simulink model "bai5"  (R2023a)
settings: Solver=VariableStepAuto  StartTime=0.0  StopTime=10.0  RelTol=1e-3
libraries: commdigbbndam3 x4, dspxfrm3 x3, eeGeneralControl x3, commchan3 x2, commsink2 x2, dspsigattribs x1, dspspect3 x1, commrflib2 x1, commrandsrc3 x1, dspstat3 x1
settings Model: Creator=USER  LastModifiedBy=Admin

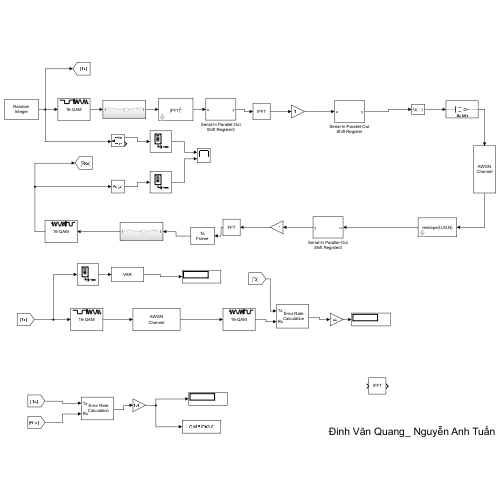
[thumbnail: Simulink's stored preview of the top-level diagram]
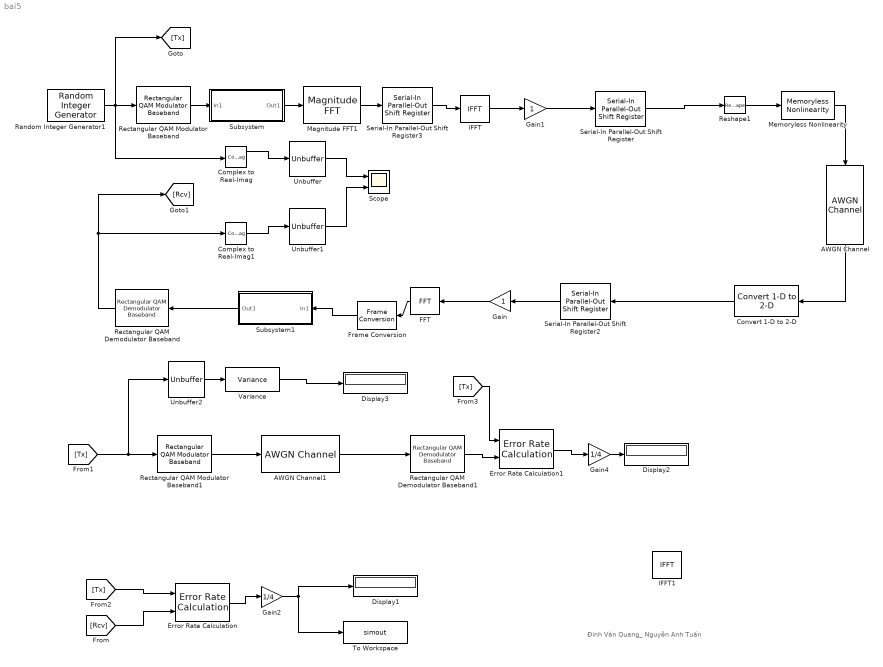
== system bai5 ==
  note: Đinh Văn Quang_ Nguyễn Anh Tuấn
  AWGN Channel : commchan3/AWGN Channel  LegacyMode=off  NoiseMethod="Signal to noise ratio  (SNR)"  noiseMode="Signal to noise ratio  (SNR)"  EbNo=10  EsNo=10  SNR=10*log10(4)  BitsPerSymbol=1  SignalPower=1  SamplesPerSymbol=1  SymbolPeriod=1  VarianceSource=Parameter  Variance=1  RandomStream=Global stream  Seed=67  SimulateUsing=Code generation
  AWGN Channel1 : commchan3/AWGN Channel  LegacyMode=off  NoiseMethod="Signal to noise ratio  (SNR)"  noiseMode="Signal to noise ratio  (SNR)"  EbNo=10  EsNo=10  SNR=10  BitsPerSymbol=1  SignalPower=1  SamplesPerSymbol=1  SymbolPeriod=1  VarianceSource=Parameter  Variance=1  RandomStream=Global stream  Seed=67  SimulateUsing=Code generation
  Complex to Real-Imag : ComplexToRealImag
  Complex to Real-Imag1 : ComplexToRealImag  Output=Real
  Convert 1-D to 2-D : dspsigattribs/Convert 1-D to 2-D  M=1  N=1  frameBasedOut=off
  Display1 : Display
  Display2 : Display
  Display3 : Display
  Error Rate Calculation : commsink2/Error Rate Calculation  N=0  st_delay=0  cp_mode=Entire frame  subframe=[]  PMode=Port  WsName=ErrorVec  RsMode2=off  stop=off  numErr=100  maxBits=1e6
  Error Rate Calculation1 : commsink2/Error Rate Calculation  N=0  st_delay=0  cp_mode=Entire frame  subframe=[]  PMode=Port  WsName=ErrorVec  RsMode2=off  stop=off  numErr=100  maxBits=1e6
  FFT : dspxfrm3/FFT  FFTImplementation=Auto  CompMethod=Table lookup  TableOpt=NEW  TableOptActive=Speed  BitRevOrder=off  Normalize=off  InheritFFTLength=on  FFTLength=64  WrapInput=on  roundingMode=Floor  overflowMode=off  firstCoeffDataTypeStr=Inherit: Same word length as input  firstCoeffLastDataTypeStr=Inherit: Same word length as input  outputMin=[]  outputMax=[]
  Frame Conversion : FrameConversion
  Gain : Gain
  Gain1 : Gain
  Gain2 : Gain  Gain=1/4
  Gain4 : Gain  Gain=1/4
  IFFT : dspxfrm3/IFFT  FFTImplementation=Auto  CompMethod=Table lookup  TableOpt=NEW  TableOptActive=Speed  BitRevOrder=off  cs_in=off  Normalize=on  InheritFFTLength=on  FFTLength=64  WrapInput=on  mode=Complex  outSamplingMode=Sample based  roundingMode=Floor  overflowMode=off  firstCoeffDataTypeStr=Inherit: Same word length as input  firstCoeffLastDataTypeStr=Inherit: Same word length as input  outputMin=[]  outputMax=[]
  IFFT1 : dspxfrm3/IFFT  FFTImplementation=Auto  CompMethod=Table lookup  TableOpt=NEW  TableOptActive=Speed  BitRevOrder=off  cs_in=off  Normalize=on  InheritFFTLength=on  FFTLength=64  WrapInput=on  mode=Complex  outSamplingMode=Sample based  roundingMode=Floor  overflowMode=off  firstCoeffDataTypeStr=Inherit: Same word length as input  firstCoeffLastDataTypeStr=Inherit: Same word length as input  outputMin=[]  outputMax=[]
  Magnitude FFT1 : dspspect3/Magnitude FFT  mag_or_magsq=Magnitude squared  FFTImplementation=Auto  fftLenInherit=off  fftsize=64  WrapInput=on
  Memoryless Nonlinearity : commrflib2/Memoryless Nonlinearity  Model=Saleh  LinearGainDB=0  TOI_Type=IIP3  IIP3=Inf  OIP3=Inf  IP1dB=Inf  OP1dB=Inf  IPsat=Inf  OPsat=Inf  Table=[ -25, 5, -1; -10, 20, -2; 0, 27, 5; 5, 28, 12 ]  MagnitudeGainDB=0  Vsat=1  MagnitudeSmooth=2  PhaseGainRadian=-.45  PhaseSaturation=.88  PhaseSmooth=3.43  InputScaleDB=0  AmAmParameters=[ 1, 0.1]  AmPmParameters=[ 0.05, 0 ]  OutputScaleDB=0  ReferenceLoad=1  SimulateUsing=Code generation
  Random Integer Generator1 : commrandsrc3/Random Integer Generator  SetSize=16  SeedSource=Parameter  Seed=37  SampleTime=1  SamplesPerFrame=960  OutputDataType=double  SimulateUsing=Interpreted execution
  Rectangular QAM Demodulator Baseband : commdigbbndam3/Rectangular QAM Demodulator Baseband  M=16  OutType=Integer  DecType=Hard decision  VarSource=Dialog  Variance=1  Dec=Gray  Mapping=[0:15]  PowType=Min. distance between symbols  MinDist=2  AvgPow=1  PeakPow=1  Ph=0  outDtype1=Inherit via internal rule  outDtype2=Inherit via internal rule  derotateFactorWordLen=16  derotateFactorDataTypeStr=Inherit: Same word length as input  derotateFactorLastDataTypeStr=Inherit: Same word length as input  denormFactorWordLen=16  denormFactorDataTypeStr=Inherit: Same word length as input  denormFactorLastDataTypeStr=Inherit: Same word length as input  prodOutWordLen=32  prodOutOverflowMode=Wrap  prodOutRoundingMode=Floor  prodOutOvFlMode=off  prodOutOvFlModeLastStrValue=off  sumWordLen=32
      settings: LibrarySourceBlock=|
      | commhdldigbbndam/Rectangular QAM
      | Demodulator
      | Baseband
  Rectangular QAM Demodulator Baseband1 : commdigbbndam3/Rectangular QAM Demodulator Baseband  M=16  OutType=Integer  DecType=Hard decision  VarSource=Dialog  Variance=1  Dec=Gray  Mapping=[0:15]  PowType=Min. distance between symbols  MinDist=2  AvgPow=1  PeakPow=1  Ph=0  outDtype1=Inherit via internal rule  outDtype2=Inherit via internal rule  derotateFactorWordLen=16  derotateFactorDataTypeStr=Inherit: Same word length as input  derotateFactorLastDataTypeStr=Inherit: Same word length as input  denormFactorWordLen=16  denormFactorDataTypeStr=Inherit: Same word length as input  denormFactorLastDataTypeStr=Inherit: Same word length as input  prodOutWordLen=32  prodOutOverflowMode=Wrap  prodOutRoundingMode=Floor  prodOutOvFlMode=off  prodOutOvFlModeLastStrValue=off  sumWordLen=32
      settings: LibrarySourceBlock=|
      | commhdldigbbndam/Rectangular QAM
      | Demodulator
      | Baseband
  Rectangular QAM Modulator Baseband : commdigbbndam3/Rectangular QAM Modulator Baseband  M=16  InType=Integer  Enc=Gray  Mapping=[0:15]  PowType=Min. distance between symbols  MinDist=1  AvgPow=1  PeakPow=1  Ph=0  outDtype=double  outWordLen=16  outUDDataType=sfix(16)  outFracLenMode=Best precision  outFracLen=15  outDataTypeStr=double  outLastDataTypeStr=double
      settings: LibrarySourceBlock=|
      | commhdldigbbndam/Rectangular QAM
      | Modulator
      | Baseband
  Rectangular QAM Modulator Baseband1 : commdigbbndam3/Rectangular QAM Modulator Baseband  M=16  InType=Integer  Enc=Gray  Mapping=[0:15]  PowType=Min. distance between symbols  MinDist=2  AvgPow=1  PeakPow=1  Ph=0  outDtype=double  outWordLen=16  outUDDataType=sfix(16)  outFracLenMode=Best precision  outFracLen=15  outDataTypeStr=double  outLastDataTypeStr=double
      settings: LibrarySourceBlock=|
      | commhdldigbbndam/Rectangular QAM
      | Modulator
      | Baseband
  Reshape1 : Reshape
  Scope : Scope  NumInputPorts=2
  Serial-In Parallel-Out Shift Register : eeGeneralControl/Serial-In Parallel-Out Shift Register  N=2  IC=0  Ts=-1
      settings: LibrarySourceBlock=|
      | ee_sl_lib/General Control/Serial-In Parallel-Out
      | Shift Register
  Serial-In Parallel-Out Shift Register2 : eeGeneralControl/Serial-In Parallel-Out Shift Register  N=2  IC=0  Ts=-1
      settings: LibrarySourceBlock=|
      | ee_sl_lib/General Control/Serial-In Parallel-Out
      | Shift Register
  Serial-In Parallel-Out Shift Register3 : eeGeneralControl/Serial-In Parallel-Out Shift Register  N=4  IC=0  Ts=-1
      settings: LibrarySourceBlock=|
      | ee_sl_lib/General Control/Serial-In Parallel-Out
      | Shift Register
  Subsystem : Subsystem
  Subsystem1 : Subsystem
  To Workspace : ToWorkspace  VariableName=simout  SaveFormat=Timeseries  SampleTime=-1
  Unbuffer : Unbuffer
  Unbuffer1 : Unbuffer
  Unbuffer2 : Unbuffer
  Variance : dspstat3/Variance  run=off  InputProcessing=Columns as channels (frame based)  reset_popup=None  directionMode=Each column  dimension=1  roiEnable=off  roiType=Rectangles  roiPortion=Entire ROI  roiOutput=Individual statistics for each ROI  roiFlag=off  roundingMode=Floor  overflowMode=off
  wires:
  Random Integer Generator1/1 -> [Tx], Complex to Real-Imag/1, Rectangular QAM Modulator Baseband/1
  Rectangular QAM Modulator Baseband/1 -> Subsystem/1(In1)
  Subsystem/1(Out1) -> Magnitude FFT1/1
  IFFT/1 -> Gain1/1
  Gain1/1 -> Serial-In Parallel-Out Shift Register/1
  Serial-In Parallel-Out Shift Register/1 -> Reshape1/1
  Reshape1/1 -> Memoryless Nonlinearity/1
  Memoryless Nonlinearity/1 -> AWGN Channel/1
  Serial-In Parallel-Out Shift Register2/1 -> Gain/1
  Gain/1 -> FFT/1
  Subsystem1/1(Out1) -> Rectangular QAM Demodulator Baseband/1
  Rectangular QAM Demodulator Baseband/1 -> Complex to Real-Imag1/1, [Rcv]
  Complex to Real-Imag1/1 -> Unbuffer1/1
  Complex to Real-Imag/1 -> Unbuffer/1
  Unbuffer/1 -> Scope/1
  Unbuffer1/1 -> Scope/2
  [Tx] -> Unbuffer2/1, Rectangular QAM Modulator Baseband1/1
  Rectangular QAM Modulator Baseband1/1 -> AWGN Channel1/1
  AWGN Channel1/1 -> Rectangular QAM Demodulator Baseband1/1
  Rectangular QAM Demodulator Baseband1/1 -> Error Rate Calculation1/2
  [Tx] -> Error Rate Calculation1/1
  Error Rate Calculation1/1 -> Gain4/1
  Unbuffer2/1 -> Variance/1
  [Tx] -> Error Rate Calculation/1
  [Rcv] -> Error Rate Calculation/2
  Error Rate Calculation/1 -> Gain2/1
  Gain2/1 -> Display1/1, To Workspace/1
  Magnitude FFT1/1 -> Serial-In Parallel-Out Shift Register3/1
  Serial-In Parallel-Out Shift Register3/1 -> IFFT/1
  Variance/1 -> Display3/1
  Gain4/1 -> Display2/1
  FFT/1 -> Frame Conversion/1
  Frame Conversion/1 -> Subsystem1/1(In1)
  AWGN Channel/1 -> Convert 1-D to 2-D/1
  Convert 1-D to 2-D/1 -> Serial-In Parallel-Out Shift Register2/1

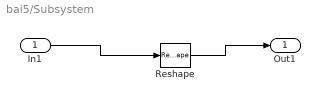
== system bai5/Subsystem ==
  In1 : Inport
  Reshape : Reshape  OutputDimensionality=Customize  OutputDimensions=[48,20]
  Out1 : Outport
  wires:
  In1/1 -> Reshape/1
  Reshape/1 -> Out1/1

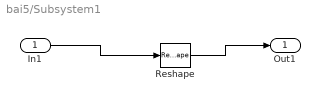
== system bai5/Subsystem1 ==
  In1 : Inport
  Reshape : Reshape  OutputDimensionality=Customize  OutputDimensions=[960,1]
  Out1 : Outport
  wires:
  In1/1 -> Reshape/1
  Reshape/1 -> Out1/1
